simulink model "model"  (R2022a)
settings: Solver=VariableStepAuto  StartTime=0.0  StopTime=10.0  RelTol=1e-3
values from neighbouring files (symbols this model uses):
  Fm = [0; 0; m*g;0;0;0]    [constants.m]
  g = 9.81    [constants.m]
  M = [  m*I,   m0_3x3 ... (first row only)    [constants.m]
  m = 2    [constants.m]
  m0_3x3 = [0,0,0; 0,0,0; 0,0,0]    [constants.m]
settings Model: Creator=danfo  LastModifiedBy=danfo

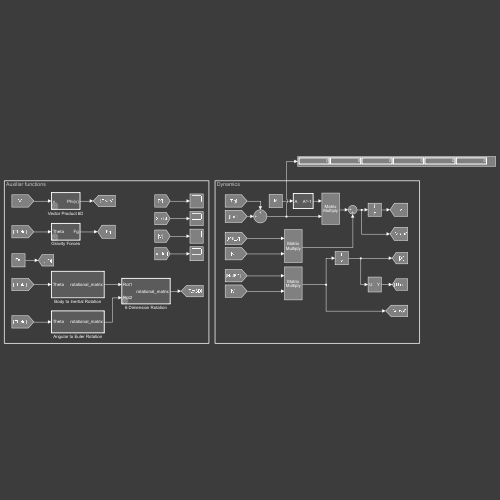
[thumbnail: Simulink's stored preview of the top-level diagram]
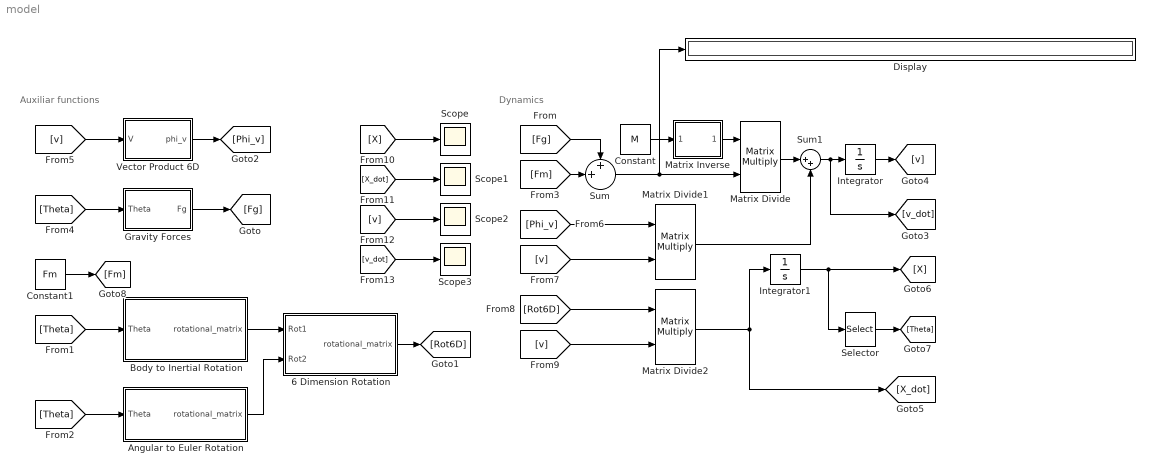
== system model ==
  note: Auxiliar functions
  note: Dynamics
  6 Dimension Rotation : MATLAB Function  TreatAsAtomicUnit=on  mask{m0_3x3=0}
  Angular to Euler Rotation : MATLAB Function  TreatAsAtomicUnit=on
  Body to Inertial Rotation : MATLAB Function  TreatAsAtomicUnit=on
  Constant : Constant  Value=M
  Constant1 : Constant  Value=Fm  VectorParams1D=off
  Display : Display
  Gravity Forces : MATLAB Function  TreatAsAtomicUnit=on  mask{m=m, g=g}
  Integrator : Integrator  InitialCondition=[0;0;0;0;0;0]
  Integrator1 : Integrator  InitialCondition=[0;0;0;0;0;0]
  Matrix Divide : Product  Inputs=**  Multiplication=Matrix(*)
  Matrix Divide1 : Product  Inputs=**  Multiplication=Matrix(*)
  Matrix Divide2 : Product  Inputs=**  Multiplication=Matrix(*)
  Matrix Inverse : MATLAB Function  TreatAsAtomicUnit=on
  Scope{,1..3} (4 alike) : Scope
  Selector : Selector  InputPortWidth=6  IndexOptions=Index vector (dialog)  Indices=[4 5 6]  OutputSizes=1
  Sum : Sum  Inputs=++|
  Sum1 : Sum  Inputs=|++
  Vector Product 6D : MATLAB Function  TreatAsAtomicUnit=on  mask{m0_3x3=m0_3x3}
  wires:
  [Fg] -> Sum/1
  Gravity Forces/1(Fg) -> [Fg]
  [Theta] -> Body to Inertial Rotation/1(Theta)
  [Theta] -> Angular to Euler Rotation/1(Theta)
  [Fm] -> Sum/2
  6 Dimension Rotation/1(rotational_matrix) -> [Rot6D]
  Angular to Euler Rotation/1(rotational_matrix) -> 6 Dimension Rotation/2(Rot2)
  Body to Inertial Rotation/1(rotational_matrix) -> 6 Dimension Rotation/1(Rot1)
  [Theta] -> Gravity Forces/1(Theta)
  [v] -> Vector Product 6D/1(V)
  Vector Product 6D/1(phi_v) -> [Phi_v]
  [Phi_v] -> Matrix Divide1/1
  [v] -> Matrix Divide1/2
  Matrix Divide/1 -> Sum1/1
  Matrix Divide1/1 -> Sum1/2
  Sum1/1 -> Integrator/1, [v_dot]
  Integrator/1 -> [v]
  [Rot6D] -> Matrix Divide2/1
  [v] -> Matrix Divide2/2
  Matrix Divide2/1 -> Integrator1/1, [X_dot]
  Integrator1/1 -> Selector/1, [X]
  [X] -> Scope/1
  [X_dot] -> Scope1/1
  [v] -> Scope2/1
  [v_dot] -> Scope3/1
  Selector/1 -> [Theta]
  Constant1/1 -> [Fm]
  Constant/1 -> Matrix Inverse/1(Matrix)
  Matrix Inverse/1(Inverse_matrix) -> Matrix Divide/1
  Sum/1 -> Display/1, Matrix Divide/2

== matlab function model/Angular to Euler Rotation ==
  data: Theta input; rotational_matrix output
%Angular velocities to Euler angles Rotation Matrix
function rotational_matrix  = Rot2(Theta)

    theta = Theta(1); phi = Theta(2);

    rotational_matrix = [1, sin(phi)*tan(theta), cos(phi)*tan(theta);
                         0, cos(phi), -sin(phi);
                         0, sin(phi)/cos(theta), cos(phi)/cos(theta)];
end

== matlab function model/Body to Inertial Rotation ==
  data: Theta input; rotational_matrix output
%Body to inertial Rotation Matrix
function rotational_matrix  = Rot1(Theta)

    theta = Theta(1); phi = Theta(2); psi = Theta(3);

    rotational_matrix = [cos(psi)*cos(theta), -cos(phi)*sin(psi)+cos(psi)*sin(phi)*sin(theta), sin(phi)*sin(psi)+cos(phi)*cos(psi)*sin(theta);
                         cos(theta)*sin(psi), cos(phi)*cos(psi)+sin(psi)*sin(theta)*sin(phi), -cos(psi)*sin(phi)+sin(psi)*sin(theta)*cos(phi);
                        -sin(theta), cos(theta)*sin(phi), cos(theta)*cos(phi)];
end

== matlab function model/6 Dimension Rotation ==
  data: Rot1 input; rotational_matrix output; Rot2 input; m0_3x3 parameter size=3,3
%6 Dimension Rotation Matrix
function rotational_matrix  = Rot6D(Rot1, Rot2, m0_3x3)

    rotational_matrix = [ Rot1,  m0_3x3;
                         m0_3x3,  Rot2 ];

end

== matlab function model/Gravity Forces ==
  data: Theta input; Fg output; m parameter; g parameter
%6 Dimension Rotation Matrix
function Fg  = Fg(Theta, m, g)

    theta = Theta(1); phi = Theta(2);

    Fg = [    m*g*sin(theta);
         -m*g*cos(theta)*sin(phi);
         -m*g*cos(theta)*cos(phi);
                     0;
                     0;
                     0;         ];

end

== matlab function model/Vector Product 6D ==
  data: V input; phi_v output; m0_3x3 parameter size=3,3
%Transposed 6 Dimension Rotation Matrix
function phi_v  = vector_product_6d(V, m0_3x3)

    %mdlWks = get_param('HexaPID','ModelWorkspace');
    %m0_3x3 = getVariable(mdlWks, "m0_3x3");
    %m0_3x3 = getVariable('ModelWorkspace', "m0_3x3");

    p = V(1); q = V(2); r = V(3); u = V(4); v = V(5); w = V(6);

    omegaxT = [0,  r, -q;
              -r,  0,  p;
               q, -p,  0];

    vxT = [0,  w, -v;
          -w,  0,  u;
           v, -u,  0];

    phi_v = [omegaxT,   m0_3x3;
               vxT,     omegaxT];

end

== matlab function model/Matrix Inverse ==
  data: Matrix input; Inverse_matrix output
%6 Dimension Rotation Matrix
function Inverse_matrix  = Inverse(Matrix)
    Inverse_matrix = inv(Matrix);
end
